simulink model "untitled"  (R2015a)
settings: Solver=ode45  StartTime=0.0  StopTime=10.0  RelTol=1e-3
settings Model: Creator=saadc  LastModifiedBy=saadc

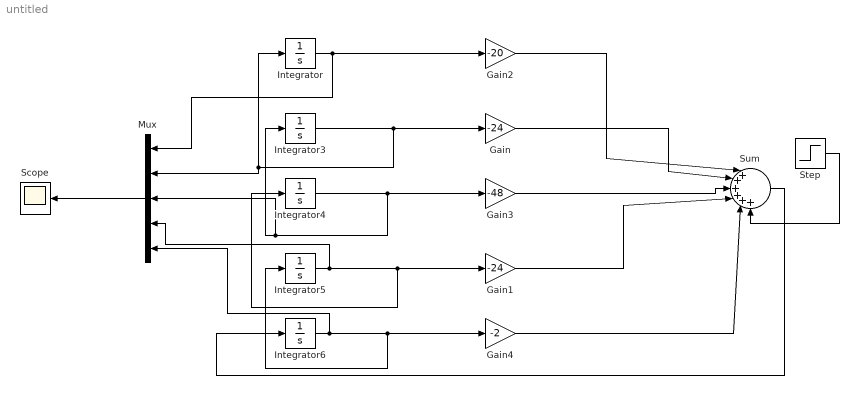
== system untitled ==
  Gain : Gain  Gain=-24
  Gain1 : Gain  Gain=-24
  Gain2 : Gain  Gain=-20
  Gain3 : Gain  Gain=-48
  Gain4 : Gain  Gain=-2
  Integrator{,3..6} (5 alike) : Integrator
  Mux : Mux  Inputs=5
  Scope : Scope
  Step : Step  After=10  SampleTime=0
  Sum : Sum  Inputs=|++++++
  wires:
  Gain2/1 -> Sum/1
  Gain/1 -> Sum/2
  Gain3/1 -> Sum/3
  Gain1/1 -> Sum/4
  Gain4/1 -> Sum/5
  Step/1 -> Sum/6
  Sum/1 -> Integrator6/1
  Integrator6/1 -> Mux/5, Gain4/1, Integrator5/1
  Integrator5/1 -> Mux/4, Integrator4/1, Gain1/1
  Integrator4/1 -> Mux/3, Integrator3/1, Gain3/1
  Integrator3/1 -> Mux/2, Integrator/1, Gain/1
  Integrator/1 -> Mux/1, Gain2/1
  Mux/1 -> Scope/1
